simulink model "AnswerC"  (R2021a)
settings: Solver=VariableStepAuto  StartTime=0.0  StopTime=10.0  RelTol=1e-3
values from neighbouring files (symbols this model uses):
  c1 = 100    [model_parameters.m]
  c2 = 1000    [model_parameters.m]
  k1 = exp(4)    [model_parameters.m]
  k2 = exp(5)    [model_parameters.m]
  m1 = 10    [model_parameters.m]
  m2 = 100    [model_parameters.m]
settings Model: Creator=jai_bhawani  LastModifiedBy=jai_bhawani

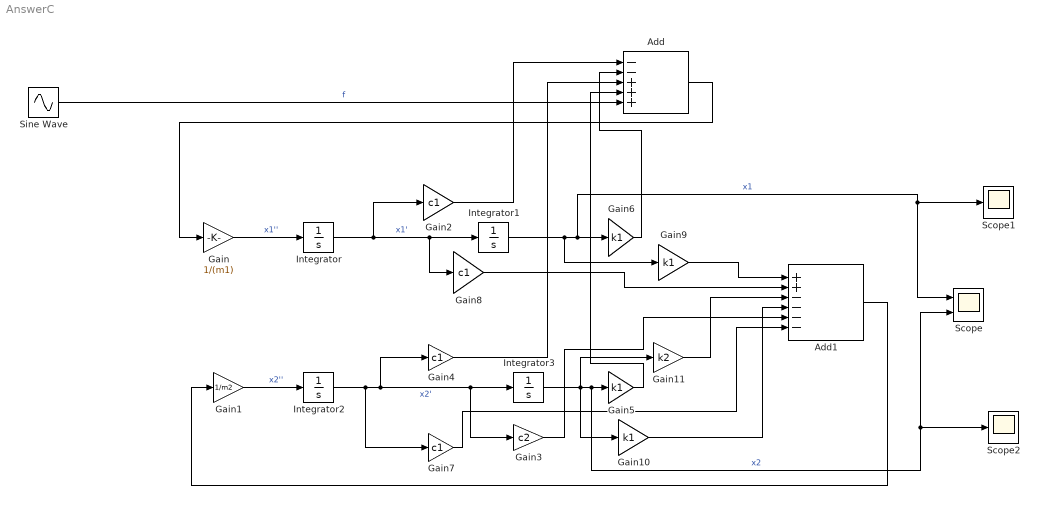
== system AnswerC ==
  Add : Sum  Inputs=--+++
  Add1 : Sum  Inputs=++----
  Gain : Gain  Gain=1/(m1)
  Gain1 : Gain  Gain=1/m2
  Gain{5..6,9..10} (4 alike) : Gain  Gain=k1
  Gain11 : Gain  Gain=k2
  Gain{2,4,7..8} (4 alike) : Gain  Gain=c1
  Gain3 : Gain  Gain=c2
  Integrator{,1..3} (4 alike) : Integrator
  Scope : Scope  NumInputPorts=2
  Scope1 : Scope
  Scope2 : Scope
  Sine Wave : Sin  Amplitude=3  Frequency=10  SampleTime=0
  wires:
  Gain/1 -> Integrator/1  "x1''"
  Gain1/1 -> Integrator2/1  "x2''"
  Integrator/1 -> Gain2/1, Integrator1/1, Gain8/1  "x1'"
  Integrator1/1 -> Gain9/1, Scope1/1, Scope/1, Gain6/1  "x1"
  Integrator2/1 -> Gain7/1, Gain4/1, Gain3/1, Integrator3/1  "x2'"
  Integrator3/1 -> Gain10/1, Scope2/1, Scope/2, Gain5/1, Gain11/1  "x2"
  Gain2/1 -> Add/1
  Gain6/1 -> Add/2
  Gain4/1 -> Add/3
  Gain5/1 -> Add/4
  Sine Wave/1 -> Add/5  "f"
  Add/1 -> Gain/1
  Gain9/1 -> Add1/1
  Gain8/1 -> Add1/2
  Gain7/1 -> Add1/6
  Gain3/1 -> Add1/5
  Gain10/1 -> Add1/4
  Gain11/1 -> Add1/3
  Add1/1 -> Gain1/1
